simulink subsystem "circle_generator"  (R2019b)
settings: Solver=VariableStepAuto  StartTime=0.0  StopTime=10.0  RelTol=1e-3
libraries: quarc_library x2, SignalEditorBlockLib x1
settings Model: Creator=icpmoles  LastModifiedBy=Student

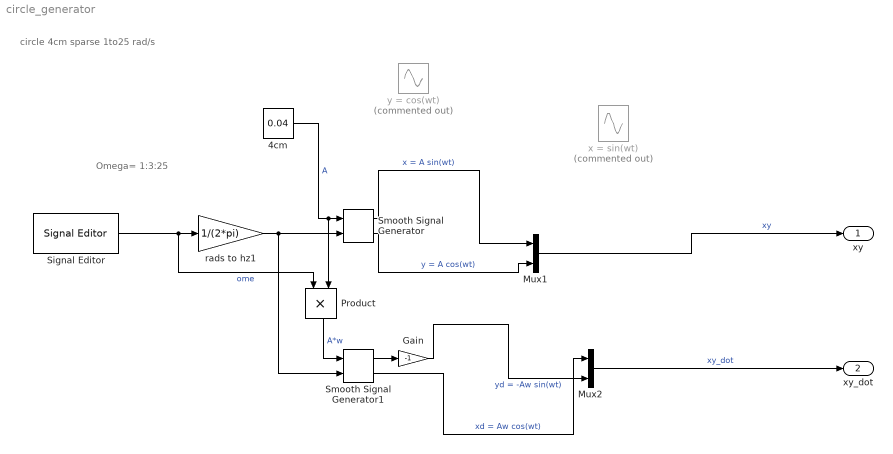
== system circle_generator ==
  note: circle 4cm sparse 1to25 rad/s
  note: Omega= 1:3:25
  4cm : Constant  Value=0.04
  Gain : Gain  Gain=-1
  Mux1 : Mux  Inputs=2
  Mux2 : Mux  Inputs=2
  Product : Product
  Signal Editor : SignalEditorBlockLib/Signal Editor  FileName=circle_omega.mat  ActiveScenario=circle  ActiveSignal=wxy  IsBus=off  OutputBusObjectStr=Bus: BusObject  SampleTime=0  Interpolate=off  ZeroCross=off  OutputAfterFinalValue=Setting to zero  Unit=inherit  PreserveSignalName=on
      settings: SourceProductName=Simulink
  Smooth Signal Generator : quarc_library/Sources/Signals/Smooth Signal Generator  signal_type=Sine  source=External (input ports)  amplitude=1  frequency=1  initial_phase=0  sample_time=qc_get_step_size  output_cos=on
      settings: SourceProductName=QUARC Targets
  Smooth Signal Generator1 : quarc_library/Sources/Signals/Smooth Signal Generator  signal_type=Sine  source=External (input ports)  amplitude=1  frequency=1  initial_phase=0  sample_time=qc_get_step_size  output_cos=on
      settings: SourceProductName=QUARC Targets
  rads to hz1 : Gain  Gain=1/(2*pi)
  x = sin(wt) : Sin  Commented=on  Amplitude=0.04  Frequency=2  SampleTime=0
  y = cos(wt) : Sin  Commented=on  Amplitude=0.04  Frequency=2  Phase=pi/2  SampleTime=0
  xy : Outport
  xy_dot : Outport  Port=2
  wires:
  Gain/1 -> Mux2/2  "yd = -Aw sin(wt)"
  Product/1 -> Smooth Signal Generator1/1  "A*w"
  Smooth Signal Generator1/2 -> Mux2/1  "xd = Aw cos(wt)"
  Smooth Signal Generator1/1 -> Gain/1
  Mux2/1 -> xy_dot/1  "xy_dot"
  4cm/1 -> Product/2, Smooth Signal Generator/1  "A"
  rads to hz1/1 -> Smooth Signal Generator1/2, Smooth Signal Generator/2
  Signal Editor/1 -> Product/1, rads to hz1/1  "ome"
  Mux1/1 -> xy/1  "xy"
  Smooth Signal Generator/2 -> Mux1/2  "y = A cos(wt)"
  Smooth Signal Generator/1 -> Mux1/1  "x = A sin(wt)"
